simulink model "ResearchPaper4Fig8"  (R2015b)
settings: Solver=VariableStepAuto  StartTime=0.0  StopTime=10.0  RelTol=1e-3
libraries: xbsIndex_r4 x484, commfilt2 x1, commrandsrc3 x1, commdigbbndam3 x1
(part 1 of 3)
settings Model: Creator=barna  LastModifiedBy=barna

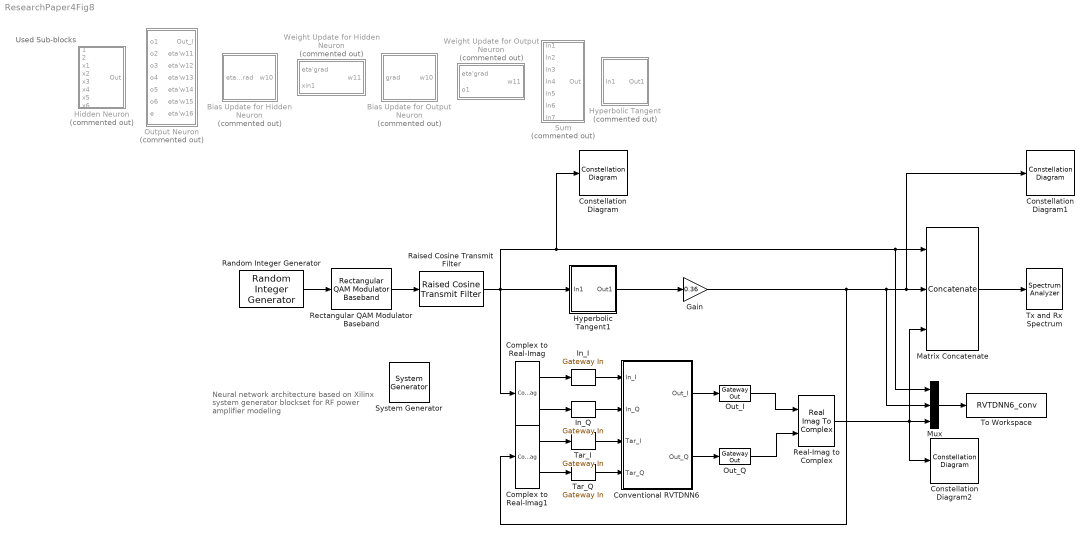
== system ResearchPaper4Fig8 ==
  note: Neural network architecture based on Xilinx system generator blockset for RF power amplifier modeling
  note: Used Sub-blocks
  " System Generator" : xbsIndex_r4/ System Generator  Tag=genX  xilinxfamily=kintex7  part=xc7k325t  speed=-3  package=fbg676  synthesis_tool=Vivado  clock_wrapper=Clock Enables  directory=./netlist  proj_type=Vivado  Synth_file=Vivado Synthesis Defaults  Impl_file=Vivado Implementation Defaults  testbench=off  simulink_period=1  sysclk_period=10  dcm_input_clock_period=10  incr_netlist=off  trim_vbits=Everywhere in SubSystem  dbl_ovrd=According to Block Masks  core_generation=According to Block Masks  run_coregen=off  deprecated_control=off  eval_field=0  block_type=sysgen
  Bias Update for Hidden Neuron : Subsystem  Commented=on
  Bias Update for Output Neuron : Subsystem  Commented=on
  Complex to Real-Imag : ComplexToRealImag
  Complex to Real-Imag1 : ComplexToRealImag
  Constellation Diagram : ConstellationDiagram
  Constellation Diagram1 : ConstellationDiagram
  Constellation Diagram2 : ConstellationDiagram
  Conventional RVTDNN6 : Subsystem
  Gain : Gain  Gain=0.36
  Hidden Neuron : Subsystem  Commented=on
  Hyperbolic Tangent : Subsystem  Commented=on
  Hyperbolic Tangent1 : Subsystem
  In_I : xbsIndex_r4/Gateway In  gui_display_data_type=Fixed-point  arith_type="Signed  (2's comp)"  n_bits=16  bin_pt=14  preci_type=Single  exp_width=8  frac_width=24  rows=1  columns=1  quantization="Round  (unbiased: +/- Inf)"  overflow=Saturate  period=1  UseAsADC=off  ADCChannel='1'  interface=None  automatic_assignment=on  address_offset=hex2dec('00')  intf_name=''  intf_description=''  default_value=0  timing_constraint=None  locs_specified=off  LOCs={}  io_standard={}  inherit_from_input=off  hdl_port=on  dbl_ovrd=off  block_type=gatewayin
  In_Q : xbsIndex_r4/Gateway In  gui_display_data_type=Fixed-point  arith_type="Signed  (2's comp)"  n_bits=16  bin_pt=14  preci_type=Single  exp_width=8  frac_width=24  rows=1  columns=1  quantization="Round  (unbiased: +/- Inf)"  overflow=Saturate  period=1  UseAsADC=off  ADCChannel='1'  interface=None  automatic_assignment=on  address_offset=hex2dec('00')  intf_name=''  intf_description=''  default_value=0  timing_constraint=None  locs_specified=off  LOCs={}  io_standard={}  inherit_from_input=off  hdl_port=on  dbl_ovrd=off  block_type=gatewayin
  Matrix Concatenate : Concatenate  NumInputs=3  Mode=Multidimensional array  ConcatenateDimension=2
  Mux : Mux  Inputs=3
  Out_I : xbsIndex_r4/Gateway Out  inherit_from_input=off  hdl_port=on  rows=1  columns=1  UseAsDAC=off  DACChannel='1'  interface=None  automatic_assignment=on  address_offset=hex2dec('00')  intf_name=''  intf_description=''  timing_constraint=None  locs_specified=off  LOCs={}  io_standard={}  block_type=gatewayout
  Out_Q : xbsIndex_r4/Gateway Out  inherit_from_input=off  hdl_port=on  rows=1  columns=1  UseAsDAC=off  DACChannel='1'  interface=None  automatic_assignment=on  address_offset=hex2dec('00')  intf_name=''  intf_description=''  timing_constraint=None  locs_specified=off  LOCs={}  io_standard={}  block_type=gatewayout
  Output Neuron : Subsystem  Commented=on
  Raised Cosine Transmit Filter : commfilt2/Raised Cosine Transmit Filter  filtType=Normal  filtSpan=20  currentFiltSpan=20  D=(20)/2  R=0.2  sampMode=Mute  saveAsFlag=0  N=20  framing=Enforce single-rate processing  InputProcessing=Columns as channels (frame based)  checkGain=Normalized  filterGain=1  checkCoeff=off  variableName=rcTxFilt  launchFVT=on  roundingMode=Floor  overflowMode=off
  Random Integer Generator : commrandsrc3/Random Integer Generator  SetSize=8  SeedSource=Auto  Seed=0  SampleTime=1  SamplesPerFrame=1  OutputDataType=double  SimulateUsing=Interpreted execution
  Real-Imag to Complex : RealImagToComplex
  Rectangular QAM Modulator Baseband : commdigbbndam3/Rectangular QAM Modulator Baseband  M=16  InType=Integer  Enc=Gray  Mapping=[0:15]  PowType=Min. distance between symbols  MinDist=2  AvgPow=1  PeakPow=1  Ph=0  outDtype=double  outWordLen=16  outUDDataType=sfix(16)  outFracLenMode=Best precision  outFracLen=15
  Sum : Subsystem  Commented=on
  Tar_I : xbsIndex_r4/Gateway In  gui_display_data_type=Fixed-point  arith_type="Signed  (2's comp)"  n_bits=16  bin_pt=14  preci_type=Single  exp_width=8  frac_width=24  rows=1  columns=1  quantization="Round  (unbiased: +/- Inf)"  overflow=Saturate  period=1  UseAsADC=off  ADCChannel='1'  interface=None  automatic_assignment=on  address_offset=hex2dec('00')  intf_name=''  intf_description=''  default_value=0  timing_constraint=None  locs_specified=off  LOCs={}  io_standard={}  inherit_from_input=off  hdl_port=on  dbl_ovrd=off  block_type=gatewayin
  Tar_Q : xbsIndex_r4/Gateway In  gui_display_data_type=Fixed-point  arith_type="Signed  (2's comp)"  n_bits=16  bin_pt=14  preci_type=Single  exp_width=8  frac_width=24  rows=1  columns=1  quantization="Round  (unbiased: +/- Inf)"  overflow=Saturate  period=1  UseAsADC=off  ADCChannel='1'  interface=None  automatic_assignment=on  address_offset=hex2dec('00')  intf_name=''  intf_description=''  default_value=0  timing_constraint=None  locs_specified=off  LOCs={}  io_standard={}  inherit_from_input=off  hdl_port=on  dbl_ovrd=off  block_type=gatewayin
  To Workspace : ToWorkspace  VariableName=RVTDNN6_conv  SaveFormat=Timeseries  SampleTime=-1
  Tx and Rx Spectrum : SpectrumAnalyzer
  Weight Update for Hidden Neuron : Subsystem  Commented=on
  Weight Update for Output Neuron : Subsystem  Commented=on
  wires:
  Random Integer Generator/1 -> Rectangular QAM Modulator Baseband/1
  Rectangular QAM Modulator Baseband/1 -> Raised Cosine Transmit Filter/1
  Complex to Real-Imag/1 -> In_I/1
  Complex to Real-Imag/2 -> In_Q/1
  Complex to Real-Imag1/1 -> Tar_I/1
  Complex to Real-Imag1/2 -> Tar_Q/1
  Out_I/1 -> Real-Imag to Complex/1
  Out_Q/1 -> Real-Imag to Complex/2
  Gain/1 -> Mux/2, Constellation Diagram1/1, Matrix Concatenate/2, Complex to Real-Imag1/1
  Raised Cosine Transmit Filter/1 -> Constellation Diagram/1, Mux/1, Matrix Concatenate/1, Hyperbolic Tangent1/1(In1), Complex to Real-Imag/1
  Real-Imag to Complex/1 -> Mux/3, Matrix Concatenate/3, Constellation Diagram2/1
  Matrix Concatenate/1 -> Tx and Rx Spectrum/1
  In_I/1 -> Conventional RVTDNN6/1(In_I)
  In_Q/1 -> Conventional RVTDNN6/2(In_Q)
  Tar_I/1 -> Conventional RVTDNN6/3(Tar_I)
  Tar_Q/1 -> Conventional RVTDNN6/4(Tar_Q)
  Conventional RVTDNN6/2(Out_Q) -> Out_Q/1
  Conventional RVTDNN6/1(Out_I) -> Out_I/1
  Hyperbolic Tangent1/1(Out1) -> Gain/1
  Mux/1 -> To Workspace/1

== system ResearchPaper4Fig8/Bias Update for Hidden Neuron ==
  eta'grad : Inport
  AddSub : xbsIndex_r4/AddSub  mode=Addition  use_carryin=off  use_carryout=off  en=off  latency=0  precision=Full  arith_type=Unsigned  n_bits=16  bin_pt=14  quantization=Truncate  overflow=Wrap  use_behavioral_HDL=off  hw_selection=Fabric  pipelined=off  dbl_ovrd=off  block_type=addsub
  Register : xbsIndex_r4/Register  init=0  rst=off  en=off  dbl_ovrd=off  block_type=register
  w10 : Outport
  wires:
  Register/1 -> w10/1, AddSub/2
  AddSub/1 -> Register/1
  eta'grad/1 -> AddSub/1

== system ResearchPaper4Fig8/Bias Update for Output Neuron ==
  grad : Inport
  AddSub : xbsIndex_r4/AddSub  mode=Addition  use_carryin=off  use_carryout=off  en=off  latency=0  precision=Full  arith_type=Unsigned  n_bits=16  bin_pt=14  quantization=Truncate  overflow=Wrap  use_behavioral_HDL=off  hw_selection=Fabric  pipelined=off  dbl_ovrd=off  block_type=addsub
  Register : xbsIndex_r4/Register  init=0  rst=off  en=off  dbl_ovrd=off  block_type=register
  w10 : Outport
  wires:
  Register/1 -> w10/1, AddSub/2
  AddSub/1 -> Register/1
  grad/1 -> AddSub/1

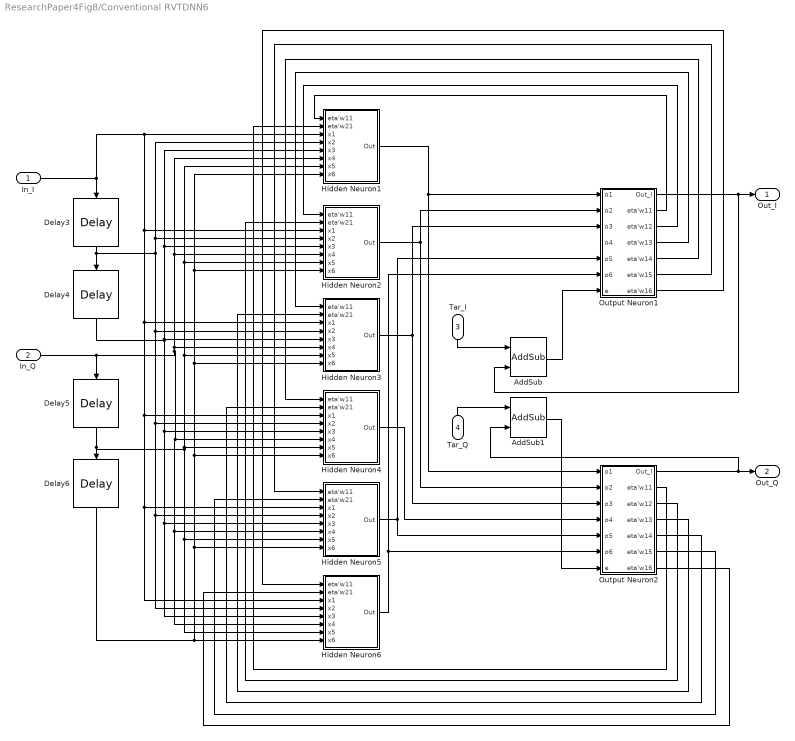
== system ResearchPaper4Fig8/Conventional RVTDNN6 ==
  In_I : Inport
  In_Q : Inport  Port=2
  Tar_I : Inport  Port=3
  Tar_Q : Inport  Port=4
  AddSub : xbsIndex_r4/AddSub  mode=Subtraction  use_carryin=off  use_carryout=off  en=off  latency=0  precision=Full  arith_type=Unsigned  n_bits=16  bin_pt=14  quantization=Truncate  overflow=Wrap  use_behavioral_HDL=off  hw_selection=Fabric  pipelined=off  dbl_ovrd=off  block_type=addsub
  AddSub1 : xbsIndex_r4/AddSub  mode=Subtraction  use_carryin=off  use_carryout=off  en=off  latency=0  precision=Full  arith_type=Unsigned  n_bits=16  bin_pt=14  quantization=Truncate  overflow=Wrap  use_behavioral_HDL=off  hw_selection=Fabric  pipelined=off  dbl_ovrd=off  block_type=addsub
  Delay{3..6} (4 alike) : xbsIndex_r4/Delay  rst=off  infoeditControl=Selection of Reset will increase slice count due to use of real FFs and instead of SRLs  en=off  latency=1  reg_retiming=off  dbl_ovrd=off  block_type=delay
  Hidden Neuron1 : Subsystem
  Hidden Neuron2 : Subsystem
  Hidden Neuron3 : Subsystem
  Hidden Neuron4 : Subsystem
  Hidden Neuron5 : Subsystem
  Hidden Neuron6 : Subsystem
  Output Neuron1 : Subsystem
  Output Neuron2 : Subsystem
  Out_I : Outport
  Out_Q : Outport  Port=2
  wires:
  Tar_I/1 -> AddSub/1
  Tar_Q/1 -> AddSub1/1
  In_Q/1 -> Hidden Neuron4/6(x4), Hidden Neuron6/6(x4), Hidden Neuron5/6(x4), Hidden Neuron3/6(x4), Hidden Neuron2/6(x4), Hidden Neuron1/6(x4), Delay5/1
  Delay5/1 -> Hidden Neuron4/7(x5), Hidden Neuron3/7(x5), Hidden Neuron2/7(x5), Hidden Neuron1/7(x5), Hidden Neuron6/7(x5), Hidden Neuron5/7(x5), Delay6/1
  Delay3/1 -> Hidden Neuron2/4(x2), Hidden Neuron1/4(x2), Hidden Neuron3/4(x2), Hidden Neuron4/4(x2), Hidden Neuron6/4(x2), Hidden Neuron5/4(x2), Delay4/1
  In_I/1 -> Hidden Neuron1/3(x1), Hidden Neuron2/3(x1), Hidden Neuron3/3(x1), Hidden Neuron4/3(x1), Hidden Neuron6/3(x1), Hidden Neuron5/3(x1), Delay3/1
  Output Neuron1/1(Out_I) -> AddSub/2, Out_I/1
  Output Neuron2/1(Out_I) -> AddSub1/2, Out_Q/1
  Output Neuron1/2(eta'w11) -> Hidden Neuron1/1(eta'w11)
  Output Neuron1/3(eta'w12) -> Hidden Neuron2/1(eta'w11)
  Output Neuron1/4(eta'w13) -> Hidden Neuron3/1(eta'w11)
  Output Neuron1/5(eta'w14) -> Hidden Neuron4/1(eta'w11)
  Output Neuron1/6(eta'w15) -> Hidden Neuron5/1(eta'w11)
  Output Neuron1/7(eta'w16) -> Hidden Neuron6/1(eta'w11)
  Output Neuron2/2(eta'w11) -> Hidden Neuron1/2(eta'w21)
  Output Neuron2/3(eta'w12) -> Hidden Neuron2/2(eta'w21)
  Output Neuron2/4(eta'w13) -> Hidden Neuron3/2(eta'w21)
  Output Neuron2/5(eta'w14) -> Hidden Neuron4/2(eta'w21)
  Output Neuron2/6(eta'w15) -> Hidden Neuron5/2(eta'w21)
  Output Neuron2/7(eta'w16) -> Hidden Neuron6/2(eta'w21)
  AddSub1/1 -> Output Neuron2/7(e)
  AddSub/1 -> Output Neuron1/7(e)
  Hidden Neuron1/1(Out) -> Output Neuron2/1(o1), Output Neuron1/1(o1)
  Hidden Neuron2/1(Out) -> Output Neuron2/2(o2), Output Neuron1/2(o2)
  Hidden Neuron3/1(Out) -> Output Neuron1/3(o3), Output Neuron2/3(o3)
  Hidden Neuron4/1(Out) -> Output Neuron2/4(o4)
  Hidden Neuron5/1(Out) -> Output Neuron2/5(o5), Output Neuron1/5(o5)
  Hidden Neuron6/1(Out) -> Output Neuron2/6(o6), Output Neuron1/6(o6)
  Delay4/1 -> Hidden Neuron3/5(x3), Hidden Neuron2/5(x3), Hidden Neuron1/5(x3), Hidden Neuron4/5(x3), Hidden Neuron6/5(x3), Hidden Neuron5/5(x3)
  Delay6/1 -> Hidden Neuron6/8(x6), Hidden Neuron5/8(x6), Hidden Neuron4/8(x6), Hidden Neuron3/8(x6), Hidden Neuron2/8(x6), Hidden Neuron1/8(x6)

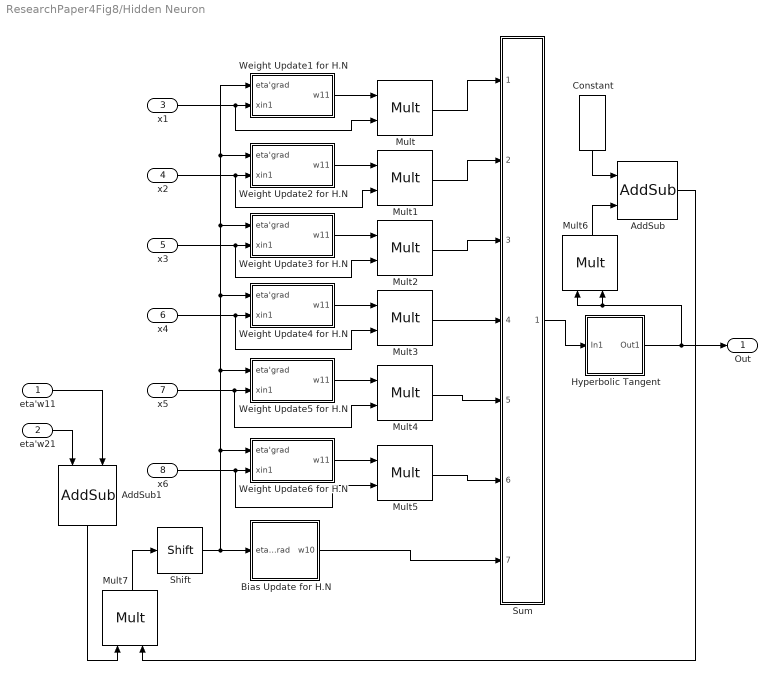
== system ResearchPaper4Fig8/Hidden Neuron ==
  eta'w11 : Inport
  eta'w21 : Inport  Port=2
  x1 : Inport  Port=3
  x2 : Inport  Port=4
  x3 : Inport  Port=5
  x4 : Inport  Port=6
  x5 : Inport  Port=7
  x6 : Inport  Port=8
  AddSub : xbsIndex_r4/AddSub  mode=Subtraction  use_carryin=off  use_carryout=off  en=off  latency=0  precision=Full  arith_type=Unsigned  n_bits=16  bin_pt=14  quantization=Truncate  overflow=Wrap  use_behavioral_HDL=off  hw_selection=Fabric  pipelined=off  dbl_ovrd=off  block_type=addsub
  AddSub1 : xbsIndex_r4/AddSub  mode=Addition  use_carryin=off  use_carryout=off  en=off  latency=0  precision=Full  arith_type=Unsigned  n_bits=16  bin_pt=14  quantization=Truncate  overflow=Wrap  use_behavioral_HDL=off  hw_selection=Fabric  pipelined=off  dbl_ovrd=off  block_type=addsub
  Bias Update for H.N : Subsystem
  Constant : xbsIndex_r4/Constant  const=1.0  gui_display_data_type=Fixed-point  arith_type=Signed (2's comp)  n_bits=16  bin_pt=14  preci_type=Single  exp_width=8  frac_width=24  explicit_period=off  period=1  equ=P=C  opselect=C  inp2=PCIN>>17  opr=+  inp1=P  carry=CIN  dbl_ovrd=off  block_type=constant
  Hyperbolic Tangent : Subsystem
  Mult{,1..7} (8 alike) : xbsIndex_r4/Mult  precision=Full  arith_type="Signed  (2's comp)"  n_bits=16  bin_pt=14  quantization=Truncate  overflow=Wrap  en=off  latency=0  use_behavioral_HDL=off  opt=Speed  use_embedded=on  optimum_pipeline=off  pipeline=on  dbl_ovrd=off  use_rpm=on  placement_style=Triangular  block_type=mult
  Shift : xbsIndex_r4/Shift  shift_dir=Right  shift_bits=4  en=off  latency=0  precision=Full  arith_type="Signed  (2's comp)"  n_bits=16  bin_pt=14  quantization=Truncate  overflow=Wrap  dbl_ovrd=off  block_type=shift
  Sum : Subsystem
  Weight Update1 for H.N : Subsystem
  Weight Update2 for H.N : Subsystem
  Weight Update3 for H.N : Subsystem
  Weight Update4 for H.N : Subsystem
  Weight Update5 for H.N : Subsystem
  Weight Update6 for H.N : Subsystem
  Out : Outport
  wires:
  Mult7/1 -> Shift/1
  Constant/1 -> AddSub/1
  Shift/1 -> Weight Update6 for H.N/1(eta'grad), Weight Update5 for H.N/1(eta'grad), Weight Update4 for H.N/1(eta'grad), Weight Update3 for H.N/1(eta'grad), Weight Update2 for H.N/1(eta'grad), Weight Update1 for H.N/1(eta'grad), Bias Update for H.N/1(eta'grad)
  Mult6/1 -> AddSub/2
  eta'w11/1 -> AddSub1/2
  Hyperbolic Tangent/1(Out1) -> Out/1, Mult6/1, Mult6/2
  AddSub1/1 -> Mult7/1
  AddSub/1 -> Mult7/2
  eta'w21/1 -> AddSub1/1
  Weight Update5 for H.N/1(w11) -> Mult4/1
  x3/1 -> Mult2/2, Weight Update3 for H.N/2(xin1)
  x5/1 -> Mult4/2, Weight Update5 for H.N/2(xin1)
  Weight Update6 for H.N/1(w11) -> Mult5/1
  Weight Update4 for H.N/1(w11) -> Mult3/1
  x2/1 -> Mult1/2, Weight Update2 for H.N/2(xin1)
  Weight Update1 for H.N/1(w11) -> Mult/1
  Weight Update2 for H.N/1(w11) -> Mult1/1
  Weight Update3 for H.N/1(w11) -> Mult2/1
  x1/1 -> Mult/2, Weight Update1 for H.N/2(xin1)
  x4/1 -> Mult3/2, Weight Update4 for H.N/2(xin1)
  x6/1 -> Mult5/2, Weight Update6 for H.N/2(xin1)
  Mult/1 -> Sum/1(In1)
  Mult1/1 -> Sum/2(In2)
  Mult2/1 -> Sum/3(In3)
  Mult3/1 -> Sum/4(In4)
  Mult4/1 -> Sum/5(In5)
  Mult5/1 -> Sum/6(In6)
  Bias Update for H.N/1(w10) -> Sum/7(In7)
  Sum/1(Out) -> Hyperbolic Tangent/1(In1)

== system ResearchPaper4Fig8/Hyperbolic Tangent ==
  In1 : Inport
  Constant : xbsIndex_r4/Constant  const=0.0  gui_display_data_type=Fixed-point  arith_type=Signed (2's comp)  n_bits=16  bin_pt=14  preci_type=Single  exp_width=8  frac_width=24  explicit_period=off  period=1  equ=P=C  opselect=C  inp2=PCIN>>17  opr=+  inp1=P  carry=CIN  dbl_ovrd=off  block_type=constant
  Mux : xbsIndex_r4/Mux  inputs=2  en=off  latency=0  precision=Full  arith_type=Unsigned  n_bits=16  bin_pt=14  quantization=Truncate  overflow=Wrap  dbl_ovrd=off  block_type=mux
  Mux1 : xbsIndex_r4/Mux  inputs=2  en=off  latency=0  precision=Full  arith_type=Unsigned  n_bits=16  bin_pt=14  quantization=Truncate  overflow=Wrap  dbl_ovrd=off  block_type=mux
  Negate : xbsIndex_r4/Negate  precision=Full  arith_type=Unsigned  n_bits=16  bin_pt=14  quantization=Truncate  overflow=Wrap  en=off  latency=0  dbl_ovrd=off  block_type=negate
  Negate1 : xbsIndex_r4/Negate  precision=Full  arith_type=Unsigned  n_bits=16  bin_pt=14  quantization=Truncate  overflow=Wrap  en=off  latency=0  dbl_ovrd=off  block_type=negate
  ROM : xbsIndex_r4/ROM  depth=16  initVector=sin(pi*(0:15)/16)  distributed_mem=Distributed memory  rst=off  init_reg=0  en=off  latency=0  gui_display_data_type=Fixed-point  arith_type="Signed  (2's comp)"  n_bits=16  bin_pt=14  preci_type=Single  exp_width=8  frac_width=24  optimize=Area  use_rpm=on  dbl_ovrd=off  block_type=sprom
  Relational : xbsIndex_r4/Relational  mode=a>b  op_type=Bool  en=off  latency=0  dbl_ovrd=off  block_type=relational
  Shift : xbsIndex_r4/Shift  shift_dir=Left  shift_bits=13  en=off  latency=0  precision=Full  arith_type="Signed  (2's comp)"  n_bits=16  bin_pt=14  quantization=Truncate  overflow=Wrap  dbl_ovrd=off  block_type=shift
  Out1 : Outport
  wires:
  Relational/1 -> Mux1/1, Mux/1
  Mux/1 -> Shift/1
  Mux1/1 -> Out1/1
  ROM/1 -> Negate1/1, Mux1/2
  Negate1/1 -> Mux1/3
  Constant/1 -> Relational/1
  In1/1 -> Negate/1, Relational/2, Mux/2
  Negate/1 -> Mux/3
  Shift/1 -> ROM/1

== system ResearchPaper4Fig8/Hyperbolic Tangent1 ==
  In1 : Inport
  Constant : xbsIndex_r4/Constant  const=0.0  gui_display_data_type=Fixed-point  arith_type=Signed (2's comp)  n_bits=16  bin_pt=14  preci_type=Single  exp_width=8  frac_width=24  explicit_period=off  period=1  equ=P=C  opselect=C  inp2=PCIN>>17  opr=+  inp1=P  carry=CIN  dbl_ovrd=off  block_type=constant
  Mux : xbsIndex_r4/Mux  inputs=2  en=off  latency=0  precision=Full  arith_type=Unsigned  n_bits=16  bin_pt=14  quantization=Truncate  overflow=Wrap  dbl_ovrd=off  block_type=mux
  Mux1 : xbsIndex_r4/Mux  inputs=2  en=off  latency=0  precision=Full  arith_type=Unsigned  n_bits=16  bin_pt=14  quantization=Truncate  overflow=Wrap  dbl_ovrd=off  block_type=mux
  Negate : xbsIndex_r4/Negate  precision=Full  arith_type=Unsigned  n_bits=16  bin_pt=14  quantization=Truncate  overflow=Wrap  en=off  latency=0  dbl_ovrd=off  block_type=negate
  Negate1 : xbsIndex_r4/Negate  precision=Full  arith_type=Unsigned  n_bits=16  bin_pt=14  quantization=Truncate  overflow=Wrap  en=off  latency=0  dbl_ovrd=off  block_type=negate
  ROM : xbsIndex_r4/ROM  depth=16  initVector=sin(pi*(0:15)/16)  distributed_mem=Distributed memory  rst=off  init_reg=0  en=off  latency=0  gui_display_data_type=Fixed-point  arith_type="Signed  (2's comp)"  n_bits=16  bin_pt=14  preci_type=Single  exp_width=8  frac_width=24  optimize=Area  use_rpm=on  dbl_ovrd=off  block_type=sprom
  Relational : xbsIndex_r4/Relational  mode=a>b  op_type=Bool  en=off  latency=0  dbl_ovrd=off  block_type=relational
  Shift : xbsIndex_r4/Shift  shift_dir=Left  shift_bits=13  en=off  latency=0  precision=Full  arith_type="Signed  (2's comp)"  n_bits=16  bin_pt=14  quantization=Truncate  overflow=Wrap  dbl_ovrd=off  block_type=shift
  Out1 : Outport
  wires:
  Relational/1 -> Mux1/1, Mux/1
  Mux/1 -> Shift/1
  Mux1/1 -> Out1/1
  ROM/1 -> Negate1/1, Mux1/2
  Negate1/1 -> Mux1/3
  Constant/1 -> Relational/1
  In1/1 -> Negate/1, Relational/2, Mux/2
  Negate/1 -> Mux/3
  Shift/1 -> ROM/1

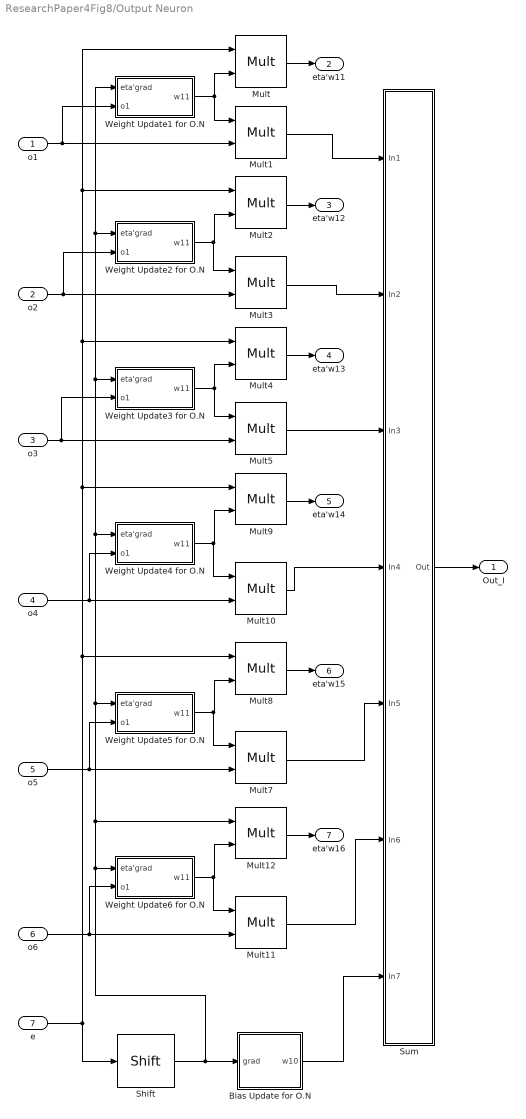
== system ResearchPaper4Fig8/Output Neuron ==
  o1 : Inport
  o2 : Inport  Port=2
  o3 : Inport  Port=3
  o4 : Inport  Port=4
  o5 : Inport  Port=5
  o6 : Inport  Port=6
  e : Inport  Port=7
  Bias Update for O.N : Subsystem
  Mult{,1..5,7..12} (12 alike) : xbsIndex_r4/Mult  precision=Full  arith_type="Signed  (2's comp)"  n_bits=16  bin_pt=14  quantization=Truncate  overflow=Wrap  en=off  latency=0  use_behavioral_HDL=off  opt=Speed  use_embedded=on  optimum_pipeline=off  pipeline=on  dbl_ovrd=off  use_rpm=on  placement_style=Triangular  block_type=mult
  Shift : xbsIndex_r4/Shift  shift_dir=Right  shift_bits=4  en=off  latency=0  precision=Full  arith_type="Signed  (2's comp)"  n_bits=16  bin_pt=14  quantization=Truncate  overflow=Wrap  dbl_ovrd=off  block_type=shift
  Sum : Subsystem
  Weight Update1 for O.N : Subsystem
  Weight Update2 for O.N : Subsystem
  Weight Update3 for O.N : Subsystem
  Weight Update4 for O.N : Subsystem
  Weight Update5 for O.N : Subsystem
  Weight Update6 for O.N : Subsystem
  Out_I : Outport
  eta'w11 : Outport  Port=2
  eta'w12 : Outport  Port=3
  eta'w13 : Outport  Port=4
  eta'w14 : Outport  Port=5
  eta'w15 : Outport  Port=6
  eta'w16 : Outport  Port=7
  wires:
  o3/1 -> Weight Update3 for O.N/2(o1), Mult5/2
  o2/1 -> Weight Update2 for O.N/2(o1), Mult3/2
  o1/1 -> Weight Update1 for O.N/2(o1), Mult1/2
  o4/1 -> Weight Update4 for O.N/2(o1), Mult10/2
  Weight Update1 for O.N/1(w11) -> Mult1/1, Mult/2
  Weight Update2 for O.N/1(w11) -> Mult3/1, Mult2/2
  Weight Update3 for O.N/1(w11) -> Mult5/1, Mult4/2
  Weight Update4 for O.N/1(w11) -> Mult10/1, Mult9/2
  Mult/1 -> eta'w11/1
  Mult2/1 -> eta'w12/1
  Mult4/1 -> eta'w13/1
  Mult9/1 -> eta'w14/1
  Mult3/1 -> Sum/2(In2)
  Shift/1 -> Weight Update6 for O.N/1(eta'grad), Mult12/1, Weight Update5 for O.N/1(eta'grad), Weight Update4 for O.N/1(eta'grad), Weight Update3 for O.N/1(eta'grad), Weight Update2 for O.N/1(eta'grad), Weight Update1 for O.N/1(eta'grad), Bias Update for O.N/1(grad)
  e/1 -> Shift/1, Mult8/1, Mult4/1, Mult2/1, Mult/1, Mult9/1
  Sum/1(Out) -> Out_I/1
  o5/1 -> Weight Update5 for O.N/2(o1), Mult7/2
  Weight Update5 for O.N/1(w11) -> Mult7/1, Mult8/2
  Mult8/1 -> eta'w15/1
  o6/1 -> Weight Update6 for O.N/2(o1), Mult11/2
  Weight Update6 for O.N/1(w11) -> Mult11/1, Mult12/2
  Mult12/1 -> eta'w16/1
  Mult1/1 -> Sum/1(In1)
  Mult5/1 -> Sum/3(In3)
  Mult10/1 -> Sum/4(In4)
  Mult7/1 -> Sum/5(In5)
  Mult11/1 -> Sum/6(In6)
  Bias Update for O.N/1(w10) -> Sum/7(In7)

== system ResearchPaper4Fig8/Sum ==
  In1 : Inport
  In2 : Inport  Port=2
  In3 : Inport  Port=3
  In4 : Inport  Port=4
  In5 : Inport  Port=5
  In6 : Inport  Port=6
  In7 : Inport  Port=7
  AddSub{,1..5} (6 alike) : xbsIndex_r4/AddSub  mode=Addition  use_carryin=off  use_carryout=off  en=off  latency=0  precision=Full  arith_type=Unsigned  n_bits=16  bin_pt=14  quantization=Truncate  overflow=Wrap  use_behavioral_HDL=off  hw_selection=Fabric  pipelined=off  dbl_ovrd=off  block_type=addsub
  Out : Outport
  wires:
  AddSub4/1 -> AddSub5/2
  AddSub3/1 -> AddSub5/1
  In7/1 -> AddSub4/2
  AddSub1/1 -> AddSub3/2
  AddSub2/1 -> AddSub4/1
  In1/1 -> AddSub/1
  In6/1 -> AddSub2/2
  In2/1 -> AddSub/2
  In4/1 -> AddSub1/2
  AddSub/1 -> AddSub3/1
  In5/1 -> AddSub2/1
  AddSub5/1 -> Out/1
  In3/1 -> AddSub1/1

== system ResearchPaper4Fig8/Weight Update for Hidden Neuron ==
  eta'grad : Inport
  xin1 : Inport  Port=2
  AddSub : xbsIndex_r4/AddSub  mode=Addition  use_carryin=off  use_carryout=off  en=off  latency=0  precision=Full  arith_type=Unsigned  n_bits=16  bin_pt=14  quantization=Truncate  overflow=Wrap  use_behavioral_HDL=off  hw_selection=Fabric  pipelined=off  dbl_ovrd=off  block_type=addsub
  Mult : xbsIndex_r4/Mult  precision=Full  arith_type="Signed  (2's comp)"  n_bits=16  bin_pt=14  quantization=Truncate  overflow=Wrap  en=off  latency=0  use_behavioral_HDL=off  opt=Speed  use_embedded=on  optimum_pipeline=off  pipeline=on  dbl_ovrd=off  use_rpm=on  placement_style=Triangular  block_type=mult
  Register : xbsIndex_r4/Register  init=0  rst=off  en=off  dbl_ovrd=off  block_type=register
  w11 : Outport
  wires:
  Mult/1 -> AddSub/1
  Register/1 -> w11/1, AddSub/2
  AddSub/1 -> Register/1
  eta'grad/1 -> Mult/1
  xin1/1 -> Mult/2

== system ResearchPaper4Fig8/Weight Update for Output Neuron ==
  eta'grad : Inport
  o1 : Inport  Port=2
  AddSub : xbsIndex_r4/AddSub  mode=Addition  use_carryin=off  use_carryout=off  en=off  latency=0  precision=Full  arith_type=Unsigned  n_bits=16  bin_pt=14  quantization=Truncate  overflow=Wrap  use_behavioral_HDL=off  hw_selection=Fabric  pipelined=off  dbl_ovrd=off  block_type=addsub
  Mult : xbsIndex_r4/Mult  precision=Full  arith_type="Signed  (2's comp)"  n_bits=16  bin_pt=14  quantization=Truncate  overflow=Wrap  en=off  latency=0  use_behavioral_HDL=off  opt=Speed  use_embedded=on  optimum_pipeline=off  pipeline=on  dbl_ovrd=off  use_rpm=on  placement_style=Triangular  block_type=mult
  Register : xbsIndex_r4/Register  init=0  rst=off  en=off  dbl_ovrd=off  block_type=register
  w11 : Outport
  wires:
  Mult/1 -> AddSub/1
  Register/1 -> w11/1, AddSub/2
  AddSub/1 -> Register/1
  eta'grad/1 -> Mult/1
  o1/1 -> Mult/2

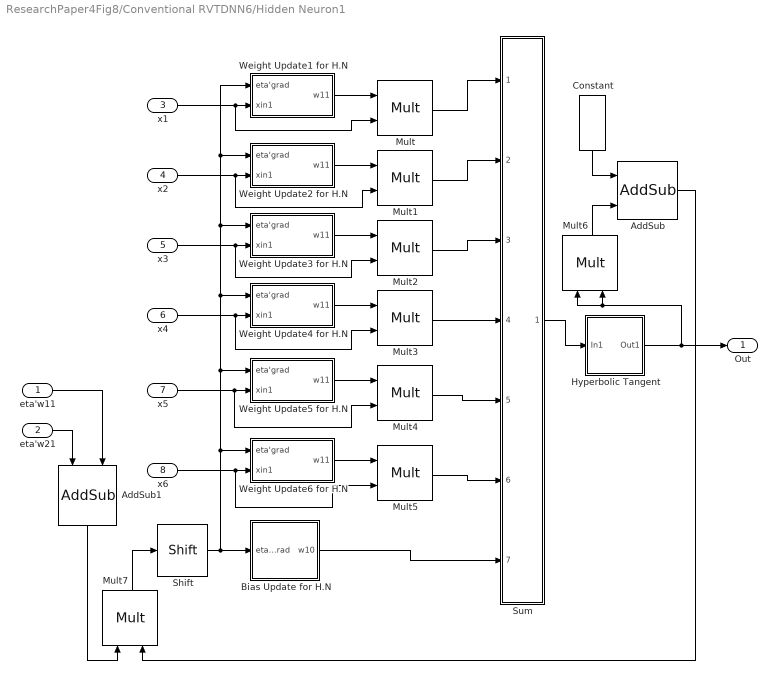
== system ResearchPaper4Fig8/Conventional RVTDNN6/Hidden Neuron1 ==
  eta'w11 : Inport
  eta'w21 : Inport  Port=2
  x1 : Inport  Port=3
  x2 : Inport  Port=4
  x3 : Inport  Port=5
  x4 : Inport  Port=6
  x5 : Inport  Port=7
  x6 : Inport  Port=8
  AddSub : xbsIndex_r4/AddSub  mode=Subtraction  use_carryin=off  use_carryout=off  en=off  latency=0  precision=Full  arith_type=Unsigned  n_bits=16  bin_pt=14  quantization=Truncate  overflow=Wrap  use_behavioral_HDL=off  hw_selection=Fabric  pipelined=off  dbl_ovrd=off  block_type=addsub
  AddSub1 : xbsIndex_r4/AddSub  mode=Addition  use_carryin=off  use_carryout=off  en=off  latency=0  precision=Full  arith_type=Unsigned  n_bits=16  bin_pt=14  quantization=Truncate  overflow=Wrap  use_behavioral_HDL=off  hw_selection=Fabric  pipelined=off  dbl_ovrd=off  block_type=addsub
  Bias Update for H.N : Subsystem
  Constant : xbsIndex_r4/Constant  const=1.0  gui_display_data_type=Fixed-point  arith_type=Signed (2's comp)  n_bits=16  bin_pt=14  preci_type=Single  exp_width=8  frac_width=24  explicit_period=off  period=1  equ=P=C  opselect=C  inp2=PCIN>>17  opr=+  inp1=P  carry=CIN  dbl_ovrd=off  block_type=constant
  Hyperbolic Tangent : Subsystem
  Mult{,1..7} (8 alike) : xbsIndex_r4/Mult  precision=Full  arith_type="Signed  (2's comp)"  n_bits=16  bin_pt=14  quantization=Truncate  overflow=Wrap  en=off  latency=0  use_behavioral_HDL=off  opt=Speed  use_embedded=on  optimum_pipeline=off  pipeline=on  dbl_ovrd=off  use_rpm=on  placement_style=Triangular  block_type=mult
  Shift : xbsIndex_r4/Shift  shift_dir=Right  shift_bits=4  en=off  latency=0  precision=Full  arith_type="Signed  (2's comp)"  n_bits=16  bin_pt=14  quantization=Truncate  overflow=Wrap  dbl_ovrd=off  block_type=shift
  Sum : Subsystem
  Weight Update1 for H.N : Subsystem
  Weight Update2 for H.N : Subsystem
  Weight Update3 for H.N : Subsystem
  Weight Update4 for H.N : Subsystem
  Weight Update5 for H.N : Subsystem
  Weight Update6 for H.N : Subsystem
  Out : Outport
  wires:
  Mult7/1 -> Shift/1
  Constant/1 -> AddSub/1
  Shift/1 -> Weight Update6 for H.N/1(eta'grad), Weight Update5 for H.N/1(eta'grad), Weight Update4 for H.N/1(eta'grad), Weight Update3 for H.N/1(eta'grad), Weight Update2 for H.N/1(eta'grad), Weight Update1 for H.N/1(eta'grad), Bias Update for H.N/1(eta'grad)
  Mult6/1 -> AddSub/2
  eta'w11/1 -> AddSub1/2
  Hyperbolic Tangent/1(Out1) -> Out/1, Mult6/1, Mult6/2
  AddSub1/1 -> Mult7/1
  AddSub/1 -> Mult7/2
  eta'w21/1 -> AddSub1/1
  Weight Update5 for H.N/1(w11) -> Mult4/1
  x3/1 -> Mult2/2, Weight Update3 for H.N/2(xin1)
  x5/1 -> Mult4/2, Weight Update5 for H.N/2(xin1)
  Weight Update6 for H.N/1(w11) -> Mult5/1
  Weight Update4 for H.N/1(w11) -> Mult3/1
  x2/1 -> Mult1/2, Weight Update2 for H.N/2(xin1)
  Weight Update1 for H.N/1(w11) -> Mult/1
  Weight Update2 for H.N/1(w11) -> Mult1/1
  Weight Update3 for H.N/1(w11) -> Mult2/1
  x1/1 -> Mult/2, Weight Update1 for H.N/2(xin1)
  x4/1 -> Mult3/2, Weight Update4 for H.N/2(xin1)
  x6/1 -> Mult5/2, Weight Update6 for H.N/2(xin1)
  Mult/1 -> Sum/1(In1)
  Mult1/1 -> Sum/2(In2)
  Mult2/1 -> Sum/3(In3)
  Mult3/1 -> Sum/4(In4)
  Mult4/1 -> Sum/5(In5)
  Mult5/1 -> Sum/6(In6)
  Bias Update for H.N/1(w10) -> Sum/7(In7)
  Sum/1(Out) -> Hyperbolic Tangent/1(In1)

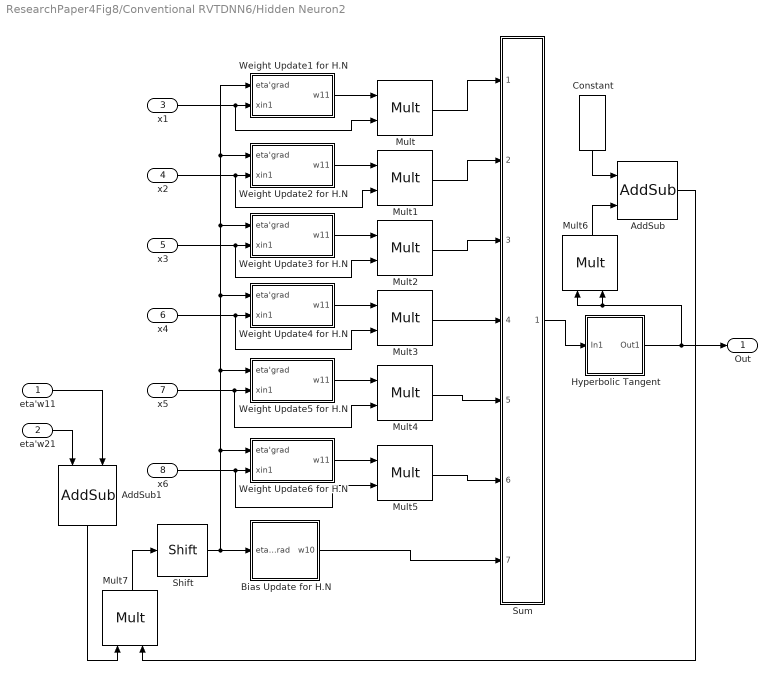
== system ResearchPaper4Fig8/Conventional RVTDNN6/Hidden Neuron2 ==
  eta'w11 : Inport
  eta'w21 : Inport  Port=2
  x1 : Inport  Port=3
  x2 : Inport  Port=4
  x3 : Inport  Port=5
  x4 : Inport  Port=6
  x5 : Inport  Port=7
  x6 : Inport  Port=8
  AddSub : xbsIndex_r4/AddSub  mode=Subtraction  use_carryin=off  use_carryout=off  en=off  latency=0  precision=Full  arith_type=Unsigned  n_bits=16  bin_pt=14  quantization=Truncate  overflow=Wrap  use_behavioral_HDL=off  hw_selection=Fabric  pipelined=off  dbl_ovrd=off  block_type=addsub
  AddSub1 : xbsIndex_r4/AddSub  mode=Addition  use_carryin=off  use_carryout=off  en=off  latency=0  precision=Full  arith_type=Unsigned  n_bits=16  bin_pt=14  quantization=Truncate  overflow=Wrap  use_behavioral_HDL=off  hw_selection=Fabric  pipelined=off  dbl_ovrd=off  block_type=addsub
  Bias Update for H.N : Subsystem
  Constant : xbsIndex_r4/Constant  const=1.0  gui_display_data_type=Fixed-point  arith_type=Signed (2's comp)  n_bits=16  bin_pt=14  preci_type=Single  exp_width=8  frac_width=24  explicit_period=off  period=1  equ=P=C  opselect=C  inp2=PCIN>>17  opr=+  inp1=P  carry=CIN  dbl_ovrd=off  block_type=constant
  Hyperbolic Tangent : Subsystem
  Mult{,1..7} (8 alike) : xbsIndex_r4/Mult  precision=Full  arith_type="Signed  (2's comp)"  n_bits=16  bin_pt=14  quantization=Truncate  overflow=Wrap  en=off  latency=0  use_behavioral_HDL=off  opt=Speed  use_embedded=on  optimum_pipeline=off  pipeline=on  dbl_ovrd=off  use_rpm=on  placement_style=Triangular  block_type=mult
  Shift : xbsIndex_r4/Shift  shift_dir=Right  shift_bits=4  en=off  latency=0  precision=Full  arith_type="Signed  (2's comp)"  n_bits=16  bin_pt=14  quantization=Truncate  overflow=Wrap  dbl_ovrd=off  block_type=shift
  Sum : Subsystem
  Weight Update1 for H.N : Subsystem
  Weight Update2 for H.N : Subsystem
  Weight Update3 for H.N : Subsystem
  Weight Update4 for H.N : Subsystem
  Weight Update5 for H.N : Subsystem
  Weight Update6 for H.N : Subsystem
  Out : Outport
  wires:
  Mult7/1 -> Shift/1
  Constant/1 -> AddSub/1
  Shift/1 -> Weight Update6 for H.N/1(eta'grad), Weight Update5 for H.N/1(eta'grad), Weight Update4 for H.N/1(eta'grad), Weight Update3 for H.N/1(eta'grad), Weight Update2 for H.N/1(eta'grad), Weight Update1 for H.N/1(eta'grad), Bias Update for H.N/1(eta'grad)
  Mult6/1 -> AddSub/2
  eta'w11/1 -> AddSub1/2
  Hyperbolic Tangent/1(Out1) -> Out/1, Mult6/1, Mult6/2
  AddSub1/1 -> Mult7/1
  AddSub/1 -> Mult7/2
  eta'w21/1 -> AddSub1/1
  Weight Update5 for H.N/1(w11) -> Mult4/1
  x3/1 -> Mult2/2, Weight Update3 for H.N/2(xin1)
  x5/1 -> Mult4/2, Weight Update5 for H.N/2(xin1)
  Weight Update6 for H.N/1(w11) -> Mult5/1
  Weight Update4 for H.N/1(w11) -> Mult3/1
  x2/1 -> Mult1/2, Weight Update2 for H.N/2(xin1)
  Weight Update1 for H.N/1(w11) -> Mult/1
  Weight Update2 for H.N/1(w11) -> Mult1/1
  Weight Update3 for H.N/1(w11) -> Mult2/1
  x1/1 -> Mult/2, Weight Update1 for H.N/2(xin1)
  x4/1 -> Mult3/2, Weight Update4 for H.N/2(xin1)
  x6/1 -> Mult5/2, Weight Update6 for H.N/2(xin1)
  Mult/1 -> Sum/1(In1)
  Mult1/1 -> Sum/2(In2)
  Mult2/1 -> Sum/3(In3)
  Mult3/1 -> Sum/4(In4)
  Mult4/1 -> Sum/5(In5)
  Mult5/1 -> Sum/6(In6)
  Bias Update for H.N/1(w10) -> Sum/7(In7)
  Sum/1(Out) -> Hyperbolic Tangent/1(In1)

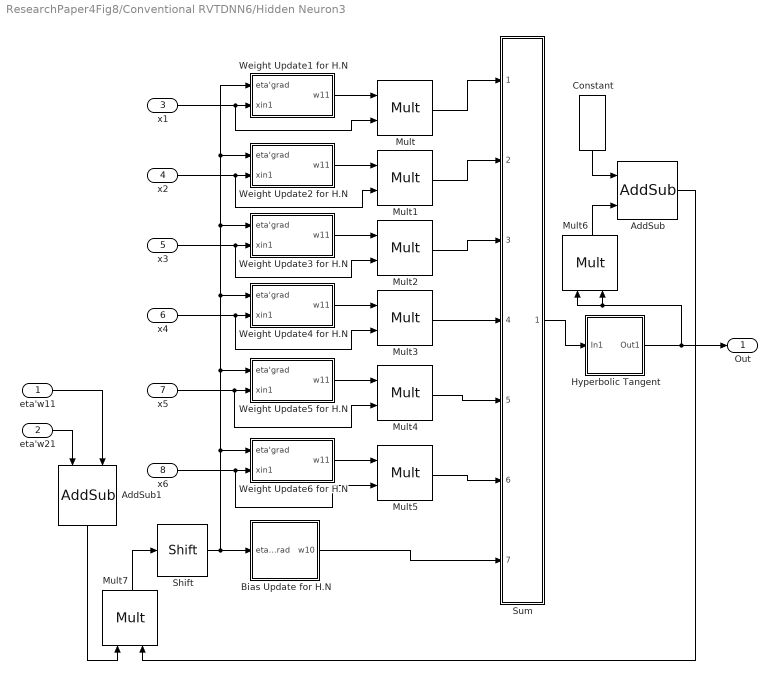
== system ResearchPaper4Fig8/Conventional RVTDNN6/Hidden Neuron3 ==
  eta'w11 : Inport
  eta'w21 : Inport  Port=2
  x1 : Inport  Port=3
  x2 : Inport  Port=4
  x3 : Inport  Port=5
  x4 : Inport  Port=6
  x5 : Inport  Port=7
  x6 : Inport  Port=8
  AddSub : xbsIndex_r4/AddSub  mode=Subtraction  use_carryin=off  use_carryout=off  en=off  latency=0  precision=Full  arith_type=Unsigned  n_bits=16  bin_pt=14  quantization=Truncate  overflow=Wrap  use_behavioral_HDL=off  hw_selection=Fabric  pipelined=off  dbl_ovrd=off  block_type=addsub
  AddSub1 : xbsIndex_r4/AddSub  mode=Addition  use_carryin=off  use_carryout=off  en=off  latency=0  precision=Full  arith_type=Unsigned  n_bits=16  bin_pt=14  quantization=Truncate  overflow=Wrap  use_behavioral_HDL=off  hw_selection=Fabric  pipelined=off  dbl_ovrd=off  block_type=addsub
  Bias Update for H.N : Subsystem
  Constant : xbsIndex_r4/Constant  const=1.0  gui_display_data_type=Fixed-point  arith_type=Signed (2's comp)  n_bits=16  bin_pt=14  preci_type=Single  exp_width=8  frac_width=24  explicit_period=off  period=1  equ=P=C  opselect=C  inp2=PCIN>>17  opr=+  inp1=P  carry=CIN  dbl_ovrd=off  block_type=constant
  Hyperbolic Tangent : Subsystem
  Mult{,1..7} (8 alike) : xbsIndex_r4/Mult  precision=Full  arith_type="Signed  (2's comp)"  n_bits=16  bin_pt=14  quantization=Truncate  overflow=Wrap  en=off  latency=0  use_behavioral_HDL=off  opt=Speed  use_embedded=on  optimum_pipeline=off  pipeline=on  dbl_ovrd=off  use_rpm=on  placement_style=Triangular  block_type=mult
  Shift : xbsIndex_r4/Shift  shift_dir=Right  shift_bits=4  en=off  latency=0  precision=Full  arith_type="Signed  (2's comp)"  n_bits=16  bin_pt=14  quantization=Truncate  overflow=Wrap  dbl_ovrd=off  block_type=shift
  Sum : Subsystem
  Weight Update1 for H.N : Subsystem
  Weight Update2 for H.N : Subsystem
  Weight Update3 for H.N : Subsystem
  Weight Update4 for H.N : Subsystem
  Weight Update5 for H.N : Subsystem
  Weight Update6 for H.N : Subsystem
  Out : Outport
  wires:
  Mult7/1 -> Shift/1
  Constant/1 -> AddSub/1
  Shift/1 -> Weight Update6 for H.N/1(eta'grad), Weight Update5 for H.N/1(eta'grad), Weight Update4 for H.N/1(eta'grad), Weight Update3 for H.N/1(eta'grad), Weight Update2 for H.N/1(eta'grad), Weight Update1 for H.N/1(eta'grad), Bias Update for H.N/1(eta'grad)
  Mult6/1 -> AddSub/2
  eta'w11/1 -> AddSub1/2
  Hyperbolic Tangent/1(Out1) -> Out/1, Mult6/1, Mult6/2
  AddSub1/1 -> Mult7/1
  AddSub/1 -> Mult7/2
  eta'w21/1 -> AddSub1/1
  Weight Update5 for H.N/1(w11) -> Mult4/1
  x3/1 -> Mult2/2, Weight Update3 for H.N/2(xin1)
  x5/1 -> Mult4/2, Weight Update5 for H.N/2(xin1)
  Weight Update6 for H.N/1(w11) -> Mult5/1
  Weight Update4 for H.N/1(w11) -> Mult3/1
  x2/1 -> Mult1/2, Weight Update2 for H.N/2(xin1)
  Weight Update1 for H.N/1(w11) -> Mult/1
  Weight Update2 for H.N/1(w11) -> Mult1/1
  Weight Update3 for H.N/1(w11) -> Mult2/1
  x1/1 -> Mult/2, Weight Update1 for H.N/2(xin1)
  x4/1 -> Mult3/2, Weight Update4 for H.N/2(xin1)
  x6/1 -> Mult5/2, Weight Update6 for H.N/2(xin1)
  Mult/1 -> Sum/1(In1)
  Mult1/1 -> Sum/2(In2)
  Mult2/1 -> Sum/3(In3)
  Mult3/1 -> Sum/4(In4)
  Mult4/1 -> Sum/5(In5)
  Mult5/1 -> Sum/6(In6)
  Bias Update for H.N/1(w10) -> Sum/7(In7)
  Sum/1(Out) -> Hyperbolic Tangent/1(In1)

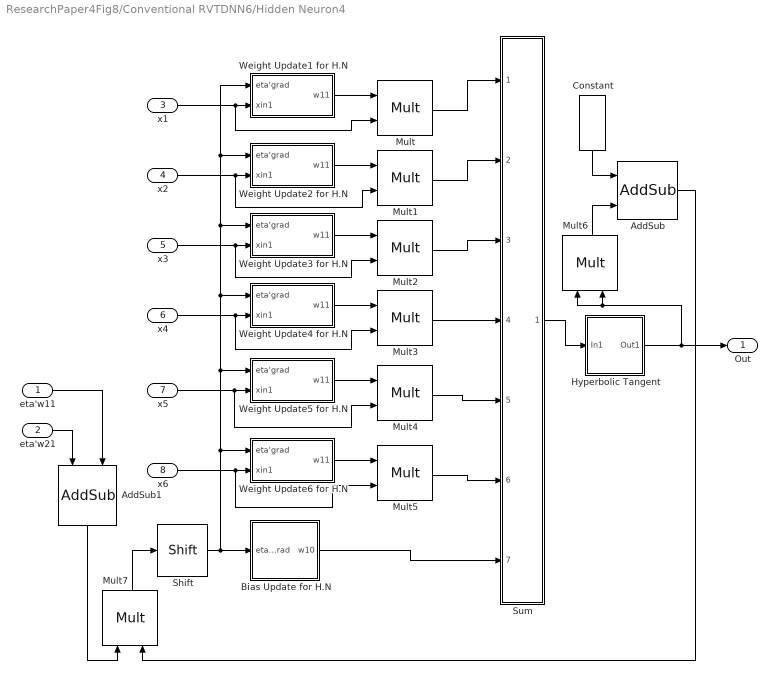
== system ResearchPaper4Fig8/Conventional RVTDNN6/Hidden Neuron4 ==
  eta'w11 : Inport
  eta'w21 : Inport  Port=2
  x1 : Inport  Port=3
  x2 : Inport  Port=4
  x3 : Inport  Port=5
  x4 : Inport  Port=6
  x5 : Inport  Port=7
  x6 : Inport  Port=8
  AddSub : xbsIndex_r4/AddSub  mode=Subtraction  use_carryin=off  use_carryout=off  en=off  latency=0  precision=Full  arith_type=Unsigned  n_bits=16  bin_pt=14  quantization=Truncate  overflow=Wrap  use_behavioral_HDL=off  hw_selection=Fabric  pipelined=off  dbl_ovrd=off  block_type=addsub
  AddSub1 : xbsIndex_r4/AddSub  mode=Addition  use_carryin=off  use_carryout=off  en=off  latency=0  precision=Full  arith_type=Unsigned  n_bits=16  bin_pt=14  quantization=Truncate  overflow=Wrap  use_behavioral_HDL=off  hw_selection=Fabric  pipelined=off  dbl_ovrd=off  block_type=addsub
  Bias Update for H.N : Subsystem
  Constant : xbsIndex_r4/Constant  const=1.0  gui_display_data_type=Fixed-point  arith_type=Signed (2's comp)  n_bits=16  bin_pt=14  preci_type=Single  exp_width=8  frac_width=24  explicit_period=off  period=1  equ=P=C  opselect=C  inp2=PCIN>>17  opr=+  inp1=P  carry=CIN  dbl_ovrd=off  block_type=constant
  Hyperbolic Tangent : Subsystem
  Mult{,1..7} (8 alike) : xbsIndex_r4/Mult  precision=Full  arith_type="Signed  (2's comp)"  n_bits=16  bin_pt=14  quantization=Truncate  overflow=Wrap  en=off  latency=0  use_behavioral_HDL=off  opt=Speed  use_embedded=on  optimum_pipeline=off  pipeline=on  dbl_ovrd=off  use_rpm=on  placement_style=Triangular  block_type=mult
  Shift : xbsIndex_r4/Shift  shift_dir=Right  shift_bits=4  en=off  latency=0  precision=Full  arith_type="Signed  (2's comp)"  n_bits=16  bin_pt=14  quantization=Truncate  overflow=Wrap  dbl_ovrd=off  block_type=shift
  Sum : Subsystem
  Weight Update1 for H.N : Subsystem
  Weight Update2 for H.N : Subsystem
  Weight Update3 for H.N : Subsystem
  Weight Update4 for H.N : Subsystem
  Weight Update5 for H.N : Subsystem
  Weight Update6 for H.N : Subsystem
  Out : Outport
  wires:
  Mult7/1 -> Shift/1
  Constant/1 -> AddSub/1
  Shift/1 -> Weight Update6 for H.N/1(eta'grad), Weight Update5 for H.N/1(eta'grad), Weight Update4 for H.N/1(eta'grad), Weight Update3 for H.N/1(eta'grad), Weight Update2 for H.N/1(eta'grad), Weight Update1 for H.N/1(eta'grad), Bias Update for H.N/1(eta'grad)
  Mult6/1 -> AddSub/2
  eta'w11/1 -> AddSub1/2
  Hyperbolic Tangent/1(Out1) -> Out/1, Mult6/1, Mult6/2
  AddSub1/1 -> Mult7/1
  AddSub/1 -> Mult7/2
  eta'w21/1 -> AddSub1/1
  Weight Update5 for H.N/1(w11) -> Mult4/1
  x3/1 -> Mult2/2, Weight Update3 for H.N/2(xin1)
  x5/1 -> Mult4/2, Weight Update5 for H.N/2(xin1)
  Weight Update6 for H.N/1(w11) -> Mult5/1
  Weight Update4 for H.N/1(w11) -> Mult3/1
  x2/1 -> Mult1/2, Weight Update2 for H.N/2(xin1)
  Weight Update1 for H.N/1(w11) -> Mult/1
  Weight Update2 for H.N/1(w11) -> Mult1/1
  Weight Update3 for H.N/1(w11) -> Mult2/1
  x1/1 -> Mult/2, Weight Update1 for H.N/2(xin1)
  x4/1 -> Mult3/2, Weight Update4 for H.N/2(xin1)
  x6/1 -> Mult5/2, Weight Update6 for H.N/2(xin1)
  Mult/1 -> Sum/1(In1)
  Mult1/1 -> Sum/2(In2)
  Mult2/1 -> Sum/3(In3)
  Mult3/1 -> Sum/4(In4)
  Mult4/1 -> Sum/5(In5)
  Mult5/1 -> Sum/6(In6)
  Bias Update for H.N/1(w10) -> Sum/7(In7)
  Sum/1(Out) -> Hyperbolic Tangent/1(In1)

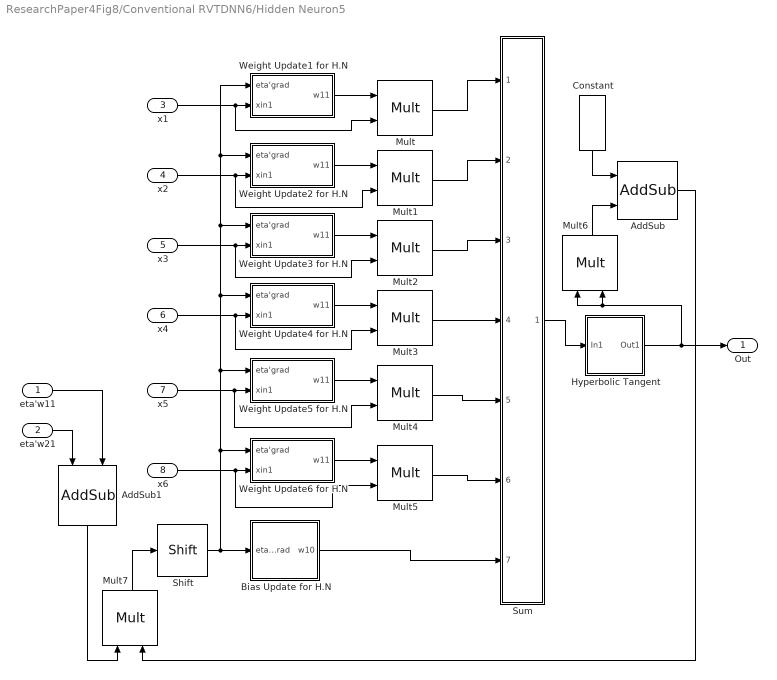
== system ResearchPaper4Fig8/Conventional RVTDNN6/Hidden Neuron5 ==
  eta'w11 : Inport
  eta'w21 : Inport  Port=2
  x1 : Inport  Port=3
  x2 : Inport  Port=4
  x3 : Inport  Port=5
  x4 : Inport  Port=6
  x5 : Inport  Port=7
  x6 : Inport  Port=8
  AddSub : xbsIndex_r4/AddSub  mode=Subtraction  use_carryin=off  use_carryout=off  en=off  latency=0  precision=Full  arith_type=Unsigned  n_bits=16  bin_pt=14  quantization=Truncate  overflow=Wrap  use_behavioral_HDL=off  hw_selection=Fabric  pipelined=off  dbl_ovrd=off  block_type=addsub
  AddSub1 : xbsIndex_r4/AddSub  mode=Addition  use_carryin=off  use_carryout=off  en=off  latency=0  precision=Full  arith_type=Unsigned  n_bits=16  bin_pt=14  quantization=Truncate  overflow=Wrap  use_behavioral_HDL=off  hw_selection=Fabric  pipelined=off  dbl_ovrd=off  block_type=addsub
  Bias Update for H.N : Subsystem
  Constant : xbsIndex_r4/Constant  const=1.0  gui_display_data_type=Fixed-point  arith_type=Signed (2's comp)  n_bits=16  bin_pt=14  preci_type=Single  exp_width=8  frac_width=24  explicit_period=off  period=1  equ=P=C  opselect=C  inp2=PCIN>>17  opr=+  inp1=P  carry=CIN  dbl_ovrd=off  block_type=constant
  Hyperbolic Tangent : Subsystem
  Mult{,1..7} (8 alike) : xbsIndex_r4/Mult  precision=Full  arith_type="Signed  (2's comp)"  n_bits=16  bin_pt=14  quantization=Truncate  overflow=Wrap  en=off  latency=0  use_behavioral_HDL=off  opt=Speed  use_embedded=on  optimum_pipeline=off  pipeline=on  dbl_ovrd=off  use_rpm=on  placement_style=Triangular  block_type=mult
  Shift : xbsIndex_r4/Shift  shift_dir=Right  shift_bits=4  en=off  latency=0  precision=Full  arith_type="Signed  (2's comp)"  n_bits=16  bin_pt=14  quantization=Truncate  overflow=Wrap  dbl_ovrd=off  block_type=shift
  Sum : Subsystem
  Weight Update1 for H.N : Subsystem
  Weight Update2 for H.N : Subsystem
  Weight Update3 for H.N : Subsystem
  Weight Update4 for H.N : Subsystem
  Weight Update5 for H.N : Subsystem
  Weight Update6 for H.N : Subsystem
  Out : Outport
  wires:
  Mult7/1 -> Shift/1
  Constant/1 -> AddSub/1
  Shift/1 -> Weight Update6 for H.N/1(eta'grad), Weight Update5 for H.N/1(eta'grad), Weight Update4 for H.N/1(eta'grad), Weight Update3 for H.N/1(eta'grad), Weight Update2 for H.N/1(eta'grad), Weight Update1 for H.N/1(eta'grad), Bias Update for H.N/1(eta'grad)
  Mult6/1 -> AddSub/2
  eta'w11/1 -> AddSub1/2
  Hyperbolic Tangent/1(Out1) -> Out/1, Mult6/1, Mult6/2
  AddSub1/1 -> Mult7/1
  AddSub/1 -> Mult7/2
  eta'w21/1 -> AddSub1/1
  Weight Update5 for H.N/1(w11) -> Mult4/1
  x3/1 -> Mult2/2, Weight Update3 for H.N/2(xin1)
  x5/1 -> Mult4/2, Weight Update5 for H.N/2(xin1)
  Weight Update6 for H.N/1(w11) -> Mult5/1
  Weight Update4 for H.N/1(w11) -> Mult3/1
  x2/1 -> Mult1/2, Weight Update2 for H.N/2(xin1)
  Weight Update1 for H.N/1(w11) -> Mult/1
  Weight Update2 for H.N/1(w11) -> Mult1/1
  Weight Update3 for H.N/1(w11) -> Mult2/1
  x1/1 -> Mult/2, Weight Update1 for H.N/2(xin1)
  x4/1 -> Mult3/2, Weight Update4 for H.N/2(xin1)
  x6/1 -> Mult5/2, Weight Update6 for H.N/2(xin1)
  Mult/1 -> Sum/1(In1)
  Mult1/1 -> Sum/2(In2)
  Mult2/1 -> Sum/3(In3)
  Mult3/1 -> Sum/4(In4)
  Mult4/1 -> Sum/5(In5)
  Mult5/1 -> Sum/6(In6)
  Bias Update for H.N/1(w10) -> Sum/7(In7)
  Sum/1(Out) -> Hyperbolic Tangent/1(In1)

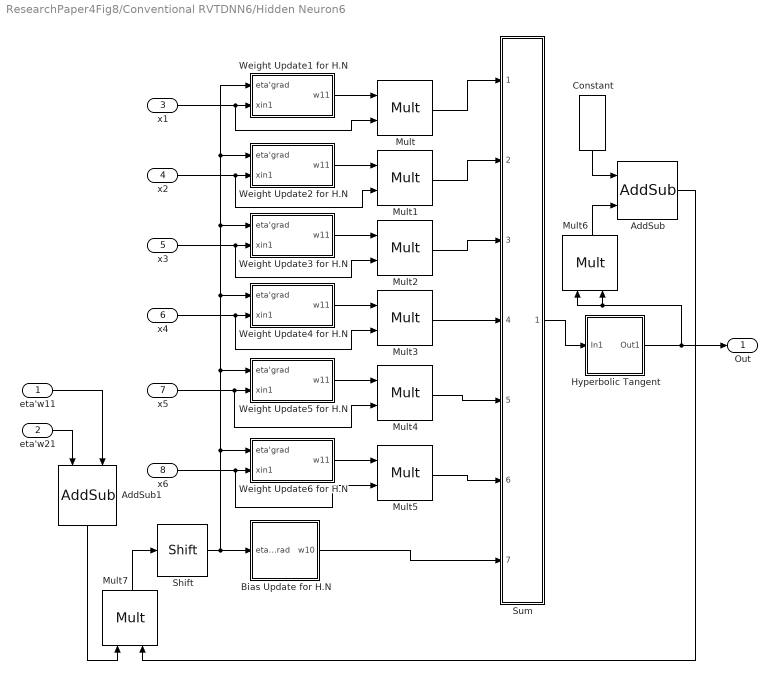
== system ResearchPaper4Fig8/Conventional RVTDNN6/Hidden Neuron6 ==
  eta'w11 : Inport
  eta'w21 : Inport  Port=2
  x1 : Inport  Port=3
  x2 : Inport  Port=4
  x3 : Inport  Port=5
  x4 : Inport  Port=6
  x5 : Inport  Port=7
  x6 : Inport  Port=8
  AddSub : xbsIndex_r4/AddSub  mode=Subtraction  use_carryin=off  use_carryout=off  en=off  latency=0  precision=Full  arith_type=Unsigned  n_bits=16  bin_pt=14  quantization=Truncate  overflow=Wrap  use_behavioral_HDL=off  hw_selection=Fabric  pipelined=off  dbl_ovrd=off  block_type=addsub
  AddSub1 : xbsIndex_r4/AddSub  mode=Addition  use_carryin=off  use_carryout=off  en=off  latency=0  precision=Full  arith_type=Unsigned  n_bits=16  bin_pt=14  quantization=Truncate  overflow=Wrap  use_behavioral_HDL=off  hw_selection=Fabric  pipelined=off  dbl_ovrd=off  block_type=addsub
  Bias Update for H.N : Subsystem
  Constant : xbsIndex_r4/Constant  const=1.0  gui_display_data_type=Fixed-point  arith_type=Signed (2's comp)  n_bits=16  bin_pt=14  preci_type=Single  exp_width=8  frac_width=24  explicit_period=off  period=1  equ=P=C  opselect=C  inp2=PCIN>>17  opr=+  inp1=P  carry=CIN  dbl_ovrd=off  block_type=constant
  Hyperbolic Tangent : Subsystem
  Mult{,1..7} (8 alike) : xbsIndex_r4/Mult  precision=Full  arith_type="Signed  (2's comp)"  n_bits=16  bin_pt=14  quantization=Truncate  overflow=Wrap  en=off  latency=0  use_behavioral_HDL=off  opt=Speed  use_embedded=on  optimum_pipeline=off  pipeline=on  dbl_ovrd=off  use_rpm=on  placement_style=Triangular  block_type=mult
  Shift : xbsIndex_r4/Shift  shift_dir=Right  shift_bits=4  en=off  latency=0  precision=Full  arith_type="Signed  (2's comp)"  n_bits=16  bin_pt=14  quantization=Truncate  overflow=Wrap  dbl_ovrd=off  block_type=shift
  Sum : Subsystem
  Weight Update1 for H.N : Subsystem
  Weight Update2 for H.N : Subsystem
  Weight Update3 for H.N : Subsystem
  Weight Update4 for H.N : Subsystem
  Weight Update5 for H.N : Subsystem
  Weight Update6 for H.N : Subsystem
  Out : Outport
  wires:
  Mult7/1 -> Shift/1
  Constant/1 -> AddSub/1
  Shift/1 -> Weight Update6 for H.N/1(eta'grad), Weight Update5 for H.N/1(eta'grad), Weight Update4 for H.N/1(eta'grad), Weight Update3 for H.N/1(eta'grad), Weight Update2 for H.N/1(eta'grad), Weight Update1 for H.N/1(eta'grad), Bias Update for H.N/1(eta'grad)
  Mult6/1 -> AddSub/2
  eta'w11/1 -> AddSub1/2
  Hyperbolic Tangent/1(Out1) -> Out/1, Mult6/1, Mult6/2
  AddSub1/1 -> Mult7/1
  AddSub/1 -> Mult7/2
  eta'w21/1 -> AddSub1/1
  Weight Update5 for H.N/1(w11) -> Mult4/1
  x3/1 -> Mult2/2, Weight Update3 for H.N/2(xin1)
  x5/1 -> Mult4/2, Weight Update5 for H.N/2(xin1)
  Weight Update6 for H.N/1(w11) -> Mult5/1
  Weight Update4 for H.N/1(w11) -> Mult3/1
  x2/1 -> Mult1/2, Weight Update2 for H.N/2(xin1)
  Weight Update1 for H.N/1(w11) -> Mult/1
  Weight Update2 for H.N/1(w11) -> Mult1/1
  Weight Update3 for H.N/1(w11) -> Mult2/1
  x1/1 -> Mult/2, Weight Update1 for H.N/2(xin1)
  x4/1 -> Mult3/2, Weight Update4 for H.N/2(xin1)
  x6/1 -> Mult5/2, Weight Update6 for H.N/2(xin1)
  Mult/1 -> Sum/1(In1)
  Mult1/1 -> Sum/2(In2)
  Mult2/1 -> Sum/3(In3)
  Mult3/1 -> Sum/4(In4)
  Mult4/1 -> Sum/5(In5)
  Mult5/1 -> Sum/6(In6)
  Bias Update for H.N/1(w10) -> Sum/7(In7)
  Sum/1(Out) -> Hyperbolic Tangent/1(In1)

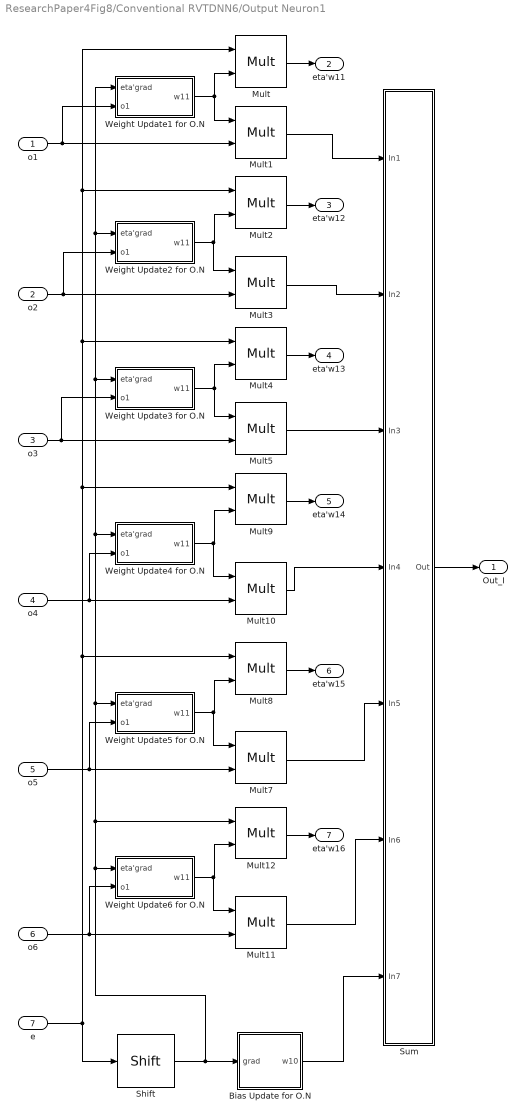
== system ResearchPaper4Fig8/Conventional RVTDNN6/Output Neuron1 ==
  o1 : Inport
  o2 : Inport  Port=2
  o3 : Inport  Port=3
  o4 : Inport  Port=4
  o5 : Inport  Port=5
  o6 : Inport  Port=6
  e : Inport  Port=7
  Bias Update for O.N : Subsystem
  Mult{,1..5,7..12} (12 alike) : xbsIndex_r4/Mult  precision=Full  arith_type="Signed  (2's comp)"  n_bits=16  bin_pt=14  quantization=Truncate  overflow=Wrap  en=off  latency=0  use_behavioral_HDL=off  opt=Speed  use_embedded=on  optimum_pipeline=off  pipeline=on  dbl_ovrd=off  use_rpm=on  placement_style=Triangular  block_type=mult
  Shift : xbsIndex_r4/Shift  shift_dir=Right  shift_bits=4  en=off  latency=0  precision=Full  arith_type="Signed  (2's comp)"  n_bits=16  bin_pt=14  quantization=Truncate  overflow=Wrap  dbl_ovrd=off  block_type=shift
  Sum : Subsystem
  Weight Update1 for O.N : Subsystem
  Weight Update2 for O.N : Subsystem
  Weight Update3 for O.N : Subsystem
  Weight Update4 for O.N : Subsystem
  Weight Update5 for O.N : Subsystem
  Weight Update6 for O.N : Subsystem
  Out_I : Outport
  eta'w11 : Outport  Port=2
  eta'w12 : Outport  Port=3
  eta'w13 : Outport  Port=4
  eta'w14 : Outport  Port=5
  eta'w15 : Outport  Port=6
  eta'w16 : Outport  Port=7
  wires:
  o3/1 -> Weight Update3 for O.N/2(o1), Mult5/2
  o2/1 -> Weight Update2 for O.N/2(o1), Mult3/2
  o1/1 -> Weight Update1 for O.N/2(o1), Mult1/2
  o4/1 -> Weight Update4 for O.N/2(o1), Mult10/2
  Weight Update1 for O.N/1(w11) -> Mult1/1, Mult/2
  Weight Update2 for O.N/1(w11) -> Mult3/1, Mult2/2
  Weight Update3 for O.N/1(w11) -> Mult5/1, Mult4/2
  Weight Update4 for O.N/1(w11) -> Mult10/1, Mult9/2
  Mult/1 -> eta'w11/1
  Mult2/1 -> eta'w12/1
  Mult4/1 -> eta'w13/1
  Mult9/1 -> eta'w14/1
  Mult3/1 -> Sum/2(In2)
  Shift/1 -> Weight Update6 for O.N/1(eta'grad), Mult12/1, Weight Update5 for O.N/1(eta'grad), Weight Update4 for O.N/1(eta'grad), Weight Update3 for O.N/1(eta'grad), Weight Update2 for O.N/1(eta'grad), Weight Update1 for O.N/1(eta'grad), Bias Update for O.N/1(grad)
  e/1 -> Shift/1, Mult8/1, Mult4/1, Mult2/1, Mult/1, Mult9/1
  Sum/1(Out) -> Out_I/1
  o5/1 -> Weight Update5 for O.N/2(o1), Mult7/2
  Weight Update5 for O.N/1(w11) -> Mult7/1, Mult8/2
  Mult8/1 -> eta'w15/1
  o6/1 -> Weight Update6 for O.N/2(o1), Mult11/2
  Weight Update6 for O.N/1(w11) -> Mult11/1, Mult12/2
  Mult12/1 -> eta'w16/1
  Mult1/1 -> Sum/1(In1)
  Mult5/1 -> Sum/3(In3)
  Mult10/1 -> Sum/4(In4)
  Mult7/1 -> Sum/5(In5)
  Mult11/1 -> Sum/6(In6)
  Bias Update for O.N/1(w10) -> Sum/7(In7)

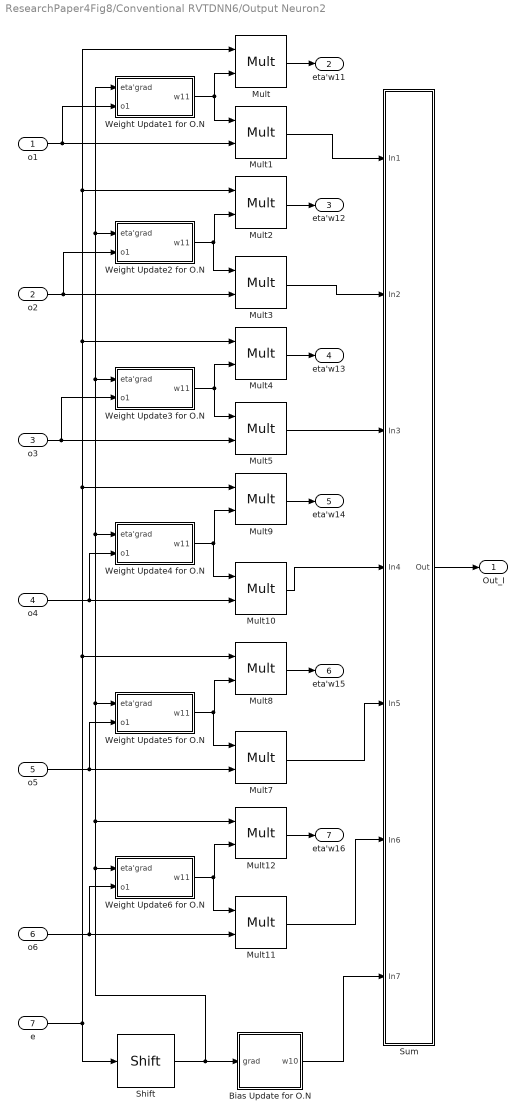
== system ResearchPaper4Fig8/Conventional RVTDNN6/Output Neuron2 ==
  o1 : Inport
  o2 : Inport  Port=2
  o3 : Inport  Port=3
  o4 : Inport  Port=4
  o5 : Inport  Port=5
  o6 : Inport  Port=6
  e : Inport  Port=7
  Bias Update for O.N : Subsystem
  Mult{,1..5,7..12} (12 alike) : xbsIndex_r4/Mult  precision=Full  arith_type="Signed  (2's comp)"  n_bits=16  bin_pt=14  quantization=Truncate  overflow=Wrap  en=off  latency=0  use_behavioral_HDL=off  opt=Speed  use_embedded=on  optimum_pipeline=off  pipeline=on  dbl_ovrd=off  use_rpm=on  placement_style=Triangular  block_type=mult
  Shift : xbsIndex_r4/Shift  shift_dir=Right  shift_bits=4  en=off  latency=0  precision=Full  arith_type="Signed  (2's comp)"  n_bits=16  bin_pt=14  quantization=Truncate  overflow=Wrap  dbl_ovrd=off  block_type=shift
  Sum : Subsystem
  Weight Update1 for O.N : Subsystem
  Weight Update2 for O.N : Subsystem
  Weight Update3 for O.N : Subsystem
  Weight Update4 for O.N : Subsystem
  Weight Update5 for O.N : Subsystem
  Weight Update6 for O.N : Subsystem
  Out_I : Outport
  eta'w11 : Outport  Port=2
  eta'w12 : Outport  Port=3
  eta'w13 : Outport  Port=4
  eta'w14 : Outport  Port=5
  eta'w15 : Outport  Port=6
  eta'w16 : Outport  Port=7
  wires:
  o3/1 -> Weight Update3 for O.N/2(o1), Mult5/2
  o2/1 -> Weight Update2 for O.N/2(o1), Mult3/2
  o1/1 -> Weight Update1 for O.N/2(o1), Mult1/2
  o4/1 -> Weight Update4 for O.N/2(o1), Mult10/2
  Weight Update1 for O.N/1(w11) -> Mult1/1, Mult/2
  Weight Update2 for O.N/1(w11) -> Mult3/1, Mult2/2
  Weight Update3 for O.N/1(w11) -> Mult5/1, Mult4/2
  Weight Update4 for O.N/1(w11) -> Mult10/1, Mult9/2
  Mult/1 -> eta'w11/1
  Mult2/1 -> eta'w12/1
  Mult4/1 -> eta'w13/1
  Mult9/1 -> eta'w14/1
  Mult3/1 -> Sum/2(In2)
  Shift/1 -> Weight Update6 for O.N/1(eta'grad), Mult12/1, Weight Update5 for O.N/1(eta'grad), Weight Update4 for O.N/1(eta'grad), Weight Update3 for O.N/1(eta'grad), Weight Update2 for O.N/1(eta'grad), Weight Update1 for O.N/1(eta'grad), Bias Update for O.N/1(grad)
  e/1 -> Shift/1, Mult8/1, Mult4/1, Mult2/1, Mult/1, Mult9/1
  Sum/1(Out) -> Out_I/1
  o5/1 -> Weight Update5 for O.N/2(o1), Mult7/2
  Weight Update5 for O.N/1(w11) -> Mult7/1, Mult8/2
  Mult8/1 -> eta'w15/1
  o6/1 -> Weight Update6 for O.N/2(o1), Mult11/2
  Weight Update6 for O.N/1(w11) -> Mult11/1, Mult12/2
  Mult12/1 -> eta'w16/1
  Mult1/1 -> Sum/1(In1)
  Mult5/1 -> Sum/3(In3)
  Mult10/1 -> Sum/4(In4)
  Mult7/1 -> Sum/5(In5)
  Mult11/1 -> Sum/6(In6)
  Bias Update for O.N/1(w10) -> Sum/7(In7)

== system ResearchPaper4Fig8/Hidden Neuron/Bias Update for H.N ==
  eta'grad : Inport
  AddSub : xbsIndex_r4/AddSub  mode=Addition  use_carryin=off  use_carryout=off  en=off  latency=0  precision=Full  arith_type=Unsigned  n_bits=16  bin_pt=14  quantization=Truncate  overflow=Wrap  use_behavioral_HDL=off  hw_selection=Fabric  pipelined=off  dbl_ovrd=off  block_type=addsub
  Register : xbsIndex_r4/Register  init=0  rst=off  en=off  dbl_ovrd=off  block_type=register
  w10 : Outport
  wires:
  Register/1 -> w10/1, AddSub/2
  AddSub/1 -> Register/1
  eta'grad/1 -> AddSub/1
